simulink library "torque_2_rpm_lib"  (R2018b)
settings: Solver=VariableStepAuto  StartTime=0.0  StopTime=10.0  RelTol=1e-3
undefined symbols (not defined in the file or in its folder): DiscIntNeverNeededParam, simParams
settings Model: Creator=Taylor  LastModifiedBy=Taylor

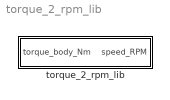
== system torque_2_rpm_lib ==
  torque_2_rpm_lib : Subsystem

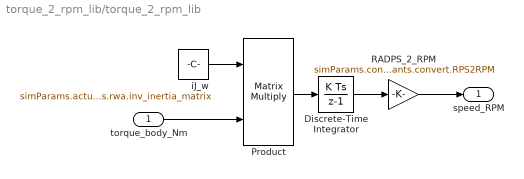
== system torque_2_rpm_lib/torque_2_rpm_lib ==
  torque_body_Nm : Inport
  Discrete-Time Integrator : DiscreteIntegrator  InitialCondition=simParams.actuators.rwa.ic.radps  SampleTime=-1  ICPrevOutput=DiscIntNeverNeededParam  ICPrevScaledInput=DiscIntNeverNeededParam
  Product : Product  Multiplication=Matrix(*)
  RADPS_2_RPM : Gain  Gain=simParams.constants.convert.RPS2RPM
  iJ_w : Constant  Value=simParams.actuators.rwa.inv_inertia_matrix
  speed_RPM : Outport
  wires:
  torque_body_Nm/1 -> Product/2
  iJ_w/1 -> Product/1
  Product/1 -> Discrete-Time Integrator/1
  Discrete-Time Integrator/1 -> RADPS_2_RPM/1
  RADPS_2_RPM/1 -> speed_RPM/1
